simulink model "BuckConverter_PowiGanControllerModeling"  (R2019a)
settings: Solver=VariableStepAuto  StartTime=0.0  StopTime=0.5  RelTol=1e-3
undefined symbols (not defined in the file): Fsw
libraries: powerlib x14, simulink x2, eePwmGenerator x1
settings Model: Creator=ryusl  LastModifiedBy=ryusl

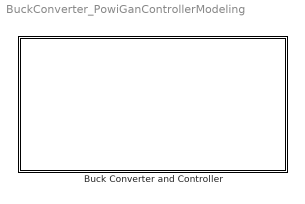
== system BuckConverter_PowiGanControllerModeling ==
  Buck Converter and Controller : Subsystem

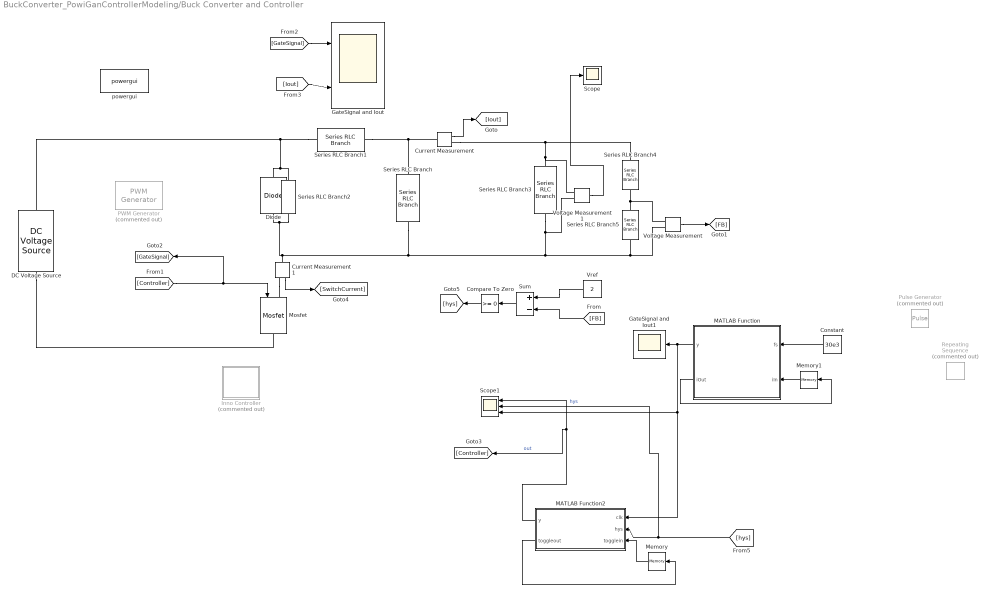
== system BuckConverter_PowiGanControllerModeling/Buck Converter and Controller ==
  Compare To Zero : simulink/Logic and Bit Operations/Compare To Zero  relop=>=  OutDataTypeStr=boolean
  Constant : Constant  Value=30e3  SampleTime=1e-6
  Current Measurement : powerlib/Measurements/Current Measurement  PhasorSimulation=off  OutputType=Complex  PSBequivalent=0
      settings: SourceProductName=Simscape Electrical
  Current Measurement1 : powerlib/Measurements/Current Measurement  PhasorSimulation=off  OutputType=Complex  PSBequivalent=0
      settings: SourceProductName=Simscape Electrical
  DC Voltage Source : powerlib/Electrical Sources/DC Voltage Source  Amplitude=100  Measurements=None
      settings: SourceProductName=Simscape Electrical
  Diode : powerlib/Power Electronics/Diode  Ron=0.001  Lon=0  Vf=0.001  IC=0  UseSnubber=0  Rs=0  Cs=0  Measurements=off
  GateSignal and Iout : Scope  NumInputPorts=2
  GateSignal and Iout1 : Scope
  Inno Controller : Stateflow chart  Commented=on  BlockKeywords=__PRM__SERIALIZED__DATA__:Stateflow Chart,Stateflow Diagram  TreatAsAtomicUnit=on
  MATLAB Function : MATLAB Function  TreatAsAtomicUnit=on
  MATLAB Function2 : MATLAB Function  TreatAsAtomicUnit=on
  Memory : Memory
  Memory1 : Memory
  Mosfet : powerlib/Power Electronics/Mosfet  Ron=0.1  Lon=0  Rd=0.01  Vfd=0.3  IC=0  Rs=500  Cs=inf  Measurements=off
  PWM Generator : eePwmGenerator/PWM Generator  Commented=on  CarrCount=Up  Tper=1/Fsw  Ts=1e-6
  Pulse Generator : DiscretePulseGenerator  Commented=on  PulseType=Time based  Period=1/(30e3)  PulseWidth=2
  Repeating Sequence : simulink/Sources/Repeating Sequence  Commented=on  rep_seq_t=[0 0.1 0.2 0.3 0.4 0.5]  rep_seq_y=[30e3 40e3 40e3 50e3 50e3 50e3]
  Scope : Scope
  Scope1 : Scope  NumInputPorts=3
  Series RLC Branch : powerlib/Elements/Series RLC Branch  LConnTagsString=__new0  RConnTagsString=__new0  BranchType=RC  Resistance=220e-3  Inductance=1e-9  SetiL0=off  InitialCurrent=0  Capacitance=68e-6  Setx0=on  InitialVoltage=24.1  Measurements=None
  Series RLC Branch1 : powerlib/Elements/Series RLC Branch  LConnTagsString=__new0  RConnTagsString=__new0  BranchType=L  Resistance=1  Inductance=1.8e-3  SetiL0=off  InitialCurrent=0  Capacitance=1e-6  Setx0=off  InitialVoltage=0  Measurements=None
  Series RLC Branch2 : powerlib/Elements/Series RLC Branch  LConnTagsString=__new0  RConnTagsString=__new0  BranchType=R  Resistance=1e6  Inductance=1e-3  SetiL0=off  InitialCurrent=0  Capacitance=1e-6  Setx0=off  InitialVoltage=0  Measurements=None
  Series RLC Branch3 : powerlib/Elements/Series RLC Branch  LConnTagsString=__new0  RConnTagsString=__new0  BranchType=R  Resistance=10  Inductance=1e-9  SetiL0=off  InitialCurrent=0  Capacitance=68e-6  Setx0=on  InitialVoltage=24.1  Measurements=None
  Series RLC Branch4 : powerlib/Elements/Series RLC Branch  LConnTagsString=__new0  RConnTagsString=__new0  BranchType=R  Resistance=11e3  Inductance=1e-9  SetiL0=off  InitialCurrent=0  Capacitance=68e-6  Setx0=on  InitialVoltage=24.1  Measurements=None
  Series RLC Branch5 : powerlib/Elements/Series RLC Branch  LConnTagsString=__new0  RConnTagsString=__new0  BranchType=R  Resistance=1e3  Inductance=1e-9  SetiL0=off  InitialCurrent=0  Capacitance=68e-6  Setx0=on  InitialVoltage=24.1  Measurements=None
  Sum : Sum  Inputs=+|-
  Voltage Measurement : powerlib/Measurements/Voltage Measurement  PhasorSimulation=off  OutputType=Complex  PSBequivalent=0
      settings: SourceProductName=Simscape Electrical
  Voltage Measurement1 : powerlib/Measurements/Voltage Measurement  PhasorSimulation=off  OutputType=Complex  PSBequivalent=0
      settings: SourceProductName=Simscape Electrical
  Vref : Constant  Value=2
  powergui : powerlib/powergui  Priority=1  SimulationMode=Discrete  SampleTime=1e-6  frequency=60  Iterations=50  frequencyindice=0  Pbase=100e6  ErrMax=1e-4  UnitsV=kV  UnitsW=MW  buscounter=0  FunctionMessages=off  echomessages=off  EnableUseOfTLC=off  CurrentSourceSwitches=off  DisableSnubberDevices=off  DisableRonSwitches=off  DisableVfSwitches=off  DisplayEquations=off  AutomaticDiscreteSolvers=off  SolverType=Tustin/Backward Euler (TBE)  Interpol=off  ExternalGateDelay=off  methode=off  Ts=100  x0status=blocks  SPID=on  SwTol=0  HookPort=off  NonlinearTolerance=0  nMaxIteration=15  ContinueOnMaxIteration=off  RestoreLinks=warning  ResistiveCurrentMeasurement=off  Frange=[0:2:500]  Ylog=off  Xlog=on  ShowGrid=off  save=off  variable=ZData  structure=0  ZoomFFT=off  StartTime=0.0  cycles=1  DisplayStyle=1  fundamental=60  FreqAxis=off  MaxFrequency=1000  frequencyindicesteady=1  RmsSteady=1  display=off
      settings: SourceProductName=Simscape Electrical
  wires:
  Current Measurement/1 -> [Iout]
  [GateSignal] -> GateSignal and Iout/1
  [Iout] -> GateSignal and Iout/2
  Voltage Measurement/1 -> [FB]
  Vref/1 -> Sum/1
  [FB] -> Sum/2
  Sum/1 -> Compare To Zero/1
  Current Measurement1/1 -> [SwitchCurrent]
  MATLAB Function2/1(y) -> [Controller], Scope1/1  "out"
  [hys] -> Scope1/2, MATLAB Function2/2(hys)  "hys"
  Compare To Zero/1 -> [hys]
  [Controller] -> [GateSignal], Mosfet/1
  Memory/1 -> MATLAB Function2/3(togglein)
  MATLAB Function2/2(toggleout) -> Memory/1
  Memory1/1 -> MATLAB Function/2(iIn)
  MATLAB Function/2(iOut) -> Memory1/1
  MATLAB Function/1(y) -> Scope1/3, MATLAB Function2/1(clk), GateSignal and Iout1/1
  Constant/1 -> MATLAB Function/1(fs)
  Voltage Measurement1/1 -> Scope/1
  connections:
  Series RLC Branch2/RConn1 -- Voltage Measurement1/LConn2 -- Series RLC Branch3/RConn1 -- Series RLC Branch5/RConn1 -- Voltage Measurement/LConn2 -- Series RLC Branch/RConn1 -- Current Measurement1/LConn1 -- Diode/LConn1
  Series RLC Branch1/RConn1 -- Current Measurement/LConn1 -- Series RLC Branch/LConn1
  Series RLC Branch1/LConn1 -- DC Voltage Source/RConn1 -- Diode/RConn1 -- Series RLC Branch2/LConn1
  DC Voltage Source/LConn1 -- Mosfet/RConn1
  Current Measurement/RConn1 -- Series RLC Branch4/LConn1 -- Voltage Measurement1/LConn1 -- Series RLC Branch3/LConn1
  Series RLC Branch5/LConn1 -- Voltage Measurement/LConn1 -- Series RLC Branch4/RConn1
  Current Measurement1/RConn1 -- Mosfet/LConn1

== matlab function BuckConverter_PowiGanControllerModeling/Buck Converter and Controller/MATLAB Function ==
  data: fs input; y output; iIn input; iOut output
function [y,iOut] = fcn(fs,iIn)
iOut = iIn;
cnt = (1/fs)/(1e-6);
cnt = int32(cnt); 
if (iIn >= cnt)
    iOut = 0;
    y = 0;
else
    if (iIn <= 2)
        y = 1;
        iOut = iOut + 1;
    else
        y = 0;
        iOut = iOut + 1;
    end
end

== stateflow chart BuckConverter_PowiGanControllerModeling/Buck Converter and Controller/Inno Controller ==
  state CheckHysteresis
    Gate = HysteresisIn;
    if (Output == HysteresisIn)
    ChangeCNT = 0;
    else
    ChangeCNT = 1;
    end
    SW = FswIn
  state SetOutput
    Output = Gate;
    if (ChangeCNT == 0 && ChangeCNT ==1)
    ChangeCNT = ChangeCNT+1;
    end
  state ControlNotChangeHysteresis
  state ControlChangeHysteresis
    if (ChangeCNT == 1)
    Output = HysteresisIn;
    ChangeCNT = 2;
    end
  (default) -> CheckHysteresis
  ControlChangeHysteresis -> CheckHysteresis : [SW ~= FswIn]
  CheckHysteresis -> SetOutput
  SetOutput -> ControlNotChangeHysteresis [order 2] : [Output == Hysteresis]
  SetOutput -> ControlChangeHysteresis [order 1] : [Output ~= HysteresisIn]

== matlab function BuckConverter_PowiGanControllerModeling/Buck Converter and Controller/MATLAB Function2 ==
  data: clk input; y output; hys input; togglein input; toggleout output
function [y,toggleout] = fcn(clk,hys,togglein)
if (clk == 1)
    y = 1;
    toggleout = 1;
else
    if (hys == 1)
        if (togglein == 0)
            y = 0;
            toggleout = 0;
        else
            y = 1;
            toggleout = 1;
        end
    else
        y = 0;
        toggleout = 0;
    end
end
